simulink model "sin_response"  (R2016a)
settings: Solver=ode5  SolverMode=SingleTasking  StartTime=0.0  StopTime=0.10  MaxStep=1/512000  RelTol=1e-3  AbsTol=1e-6
undefined symbols (not defined in the file or in its folder): DiscIntNeverNeededParam
libraries: dspmlti4 x3, dsparch4 x1
settings Model: ExtModeTrigMode=oneshot  ExtModeArmWhenConnect=off  ExtModeAutoUpdateStatusClock=off  Creator=The MathWorks, Inc.  LastModifiedBy=joa-m
settings DataIOCC: SaveFormat=Array  SaveOutput=off  SaveTime=off  SignalLoggingName=logsOut
settings OptimizationCC: BlockReduction=off  BooleanDataType=off  ExpressionDepthLimit=2147483647  RollThreshold=2  InitFltsAndDblsToZero=on  EfficientMapNaN2IntZero=off
settings DebuggingCC: SaveWithParameterizedLinksMsg=none  UnderspecifiedInitializationDetection=Classic  MergeDetectMultiDrivingBlocksExec=none  SignalResolutionControl=TryResolveAllWithWarning  MultiTaskDSMMsg=warning  MultiTaskCondExecSysMsg=none  IntegerOverflowMsg=none  FcnCallInpInsideContextMsg=UseLocalSettings  AllowSymbolicDim=off  StateNameClashWarn=warning  IntegerSaturationMsg=none
settings HardwareCC: ProdBitPerPointer=32  ProdLargestAtomicFloat=None  ProdIntDivRoundTo=Undefined  ProdEndianess=Unspecified  ProdWordSize=32  ProdHWDeviceType=32-bit Generic  TargetUnknown=on
settings ModelReferenceCC: PropagateSignalLabelsOutOfModel=off
settings GRTTargetCC: TargetFcnLib=ansi_tfl_tmw.mat  CombineOutputUpdateFcns=off  GRTInterface=on
settings ConfigComp: CovModelRefEnable=Off

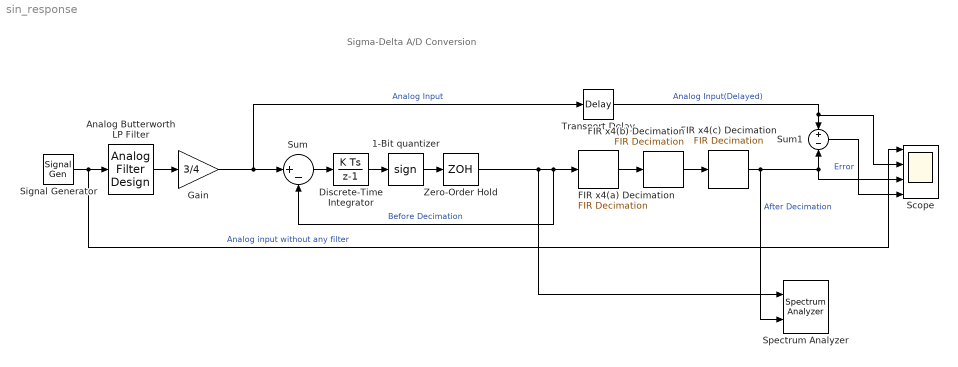
== system sin_response ==
  note: Sigma-Delta A/D Conversion
  1-Bit quantizer : Signum
  Analog Butterworth LP Filter : dsparch4/Analog Filter Design  method=Butterworth  filttype=Lowpass  N=2  Wlo=2*pi*6000  Whi=80  Rp=2  Rs=40
  Discrete-Time Integrator : DiscreteIntegrator  InitialConditionSetting=State (most efficient)  SampleTime=1/512000  ICPrevOutput=DiscIntNeverNeededParam  ICPrevScaledInput=DiscIntNeverNeededParam
  FIR x4(a) Decimation : dspmlti4/FIR Decimation  FilterSource=Dialog parameters  h=fir1(31,0.15)  D=4  filtStruct=Direct form  FilterObject=Hm_firdecim  framing=Allow multirate processing  inputOffset=0  outputBufInitCond=0  roundingMode=Floor  overflowMode=off  firstCoeffDataTypeStr=Inherit: Same word length as input  firstCoeffMin=[]  firstCoeffMax=[]  firstCoeffLastDataTypeStr=Inherit: Same word length as input  accumDataTypeStr=Inherit: Same as product output  accumLastDataTypeStr=Inherit: Same as product output  outputMin=[]  outputMax=[]
  FIR x4(b) Decimation : dspmlti4/FIR Decimation  FilterSource=Dialog parameters  h=fir1(31,0.15)  D=4  filtStruct=Direct form  FilterObject=Hm_firdecim  framing=Allow multirate processing  inputOffset=0  outputBufInitCond=0  roundingMode=Floor  overflowMode=off  firstCoeffDataTypeStr=Inherit: Same word length as input  firstCoeffMin=[]  firstCoeffMax=[]  firstCoeffLastDataTypeStr=Inherit: Same word length as input  accumDataTypeStr=Inherit: Same as product output  accumLastDataTypeStr=Inherit: Same as product output  outputMin=[]  outputMax=[]
  FIR x4(c) Decimation : dspmlti4/FIR Decimation  FilterSource=Dialog parameters  h=fir1(31,0.15)  D=4  filtStruct=Direct form  FilterObject=Hm_firdecim  framing=Allow multirate processing  inputOffset=0  outputBufInitCond=0  roundingMode=Floor  overflowMode=off  firstCoeffDataTypeStr=Inherit: Same word length as input  firstCoeffMin=[]  firstCoeffMax=[]  firstCoeffLastDataTypeStr=Inherit: Same word length as input  accumDataTypeStr=Inherit: Same as product output  accumLastDataTypeStr=Inherit: Same as product output  outputMin=[]  outputMax=[]
  Gain : Gain  Gain=3/4  SaturateOnIntegerOverflow=on  OutDataTypeStr=Inherit: Same as input  ParamDataTypeStr=Inherit: Same as input
  Scope : Scope  NumInputPorts=4
  Signal Generator : SignalGenerator  Frequency=1000
  Spectrum Analyzer : SpectrumAnalyzer  NumInputPorts=2
  Sum : Sum  Inputs=|+-  SaturateOnIntegerOverflow=on  InputSameDT=on  OutDataTypeStr=Inherit: Same as first input
  Sum1 : Sum  Inputs=+-  SaturateOnIntegerOverflow=on  InputSameDT=on  OutDataTypeStr=Inherit: Same as first input
  Transport Delay : TransportDelay  DelayTime=336/512000
  Zero-Order Hold : ZeroOrderHold  SampleTime=1/512000
  wires:
  Zero-Order Hold/1 -> Spectrum Analyzer/1, FIR x4(a) Decimation/1, Sum/2  "Before Decimation"
  1-Bit quantizer/1 -> Zero-Order Hold/1
  Sum/1 -> Discrete-Time Integrator/1
  Discrete-Time Integrator/1 -> 1-Bit quantizer/1
  FIR x4(c) Decimation/1 -> Spectrum Analyzer/2, Sum1/2, Scope/3  "After Decimation"
  Gain/1 -> Transport Delay/1, Sum/1  "Analog Input"
  Analog Butterworth LP Filter/1 -> Gain/1
  FIR x4(a) Decimation/1 -> FIR x4(b) Decimation/1
  FIR x4(b) Decimation/1 -> FIR x4(c) Decimation/1
  Transport Delay/1 -> Scope/2, Sum1/1  "Analog Input(Delayed)"
  Signal Generator/1 -> Scope/1, Analog Butterworth LP Filter/1  "Analog input without any filter"
  Sum1/1 -> Scope/4  "Error"
